simulink model "NewFSBER7f_1"  (Simulink 8.0)
settings: Solver=ode45  StartTime=0.0  StopTime=SystemSettings.SimEndTime  RelTol=1e-3
undefined symbols (not defined in the file): ChannelSettings, dfilt, outputcontrol, ShaperSettings, SystemSettings
libraries: dspmathops x14, dspsigattribs x10, dspsigops x9, simulink x5, dsparch4 x3, dspsrcs4 x3, commchan3 x1, commsink2 x1, commrandsrc2 x1
settings Model: Creator=cthomos  LastModifiedBy=Christos
settings DataIOCC: SignalLoggingSaveFormat=ModelDataLogs
settings OptimizationCC: InitFltsAndDblsToZero=on
settings DebuggingCC: SaveWithParameterizedLinksMsg=none  SignalResolutionControl=TryResolveAllWithWarning  FcnCallInpInsideContextMsg=UseLocalSettings  StrictBusMsg=Warning
settings GRTTargetCC: TargetFcnLib=ansi_tfl_tmw.mat  CombineOutputUpdateFcns=off  GRTInterface=on

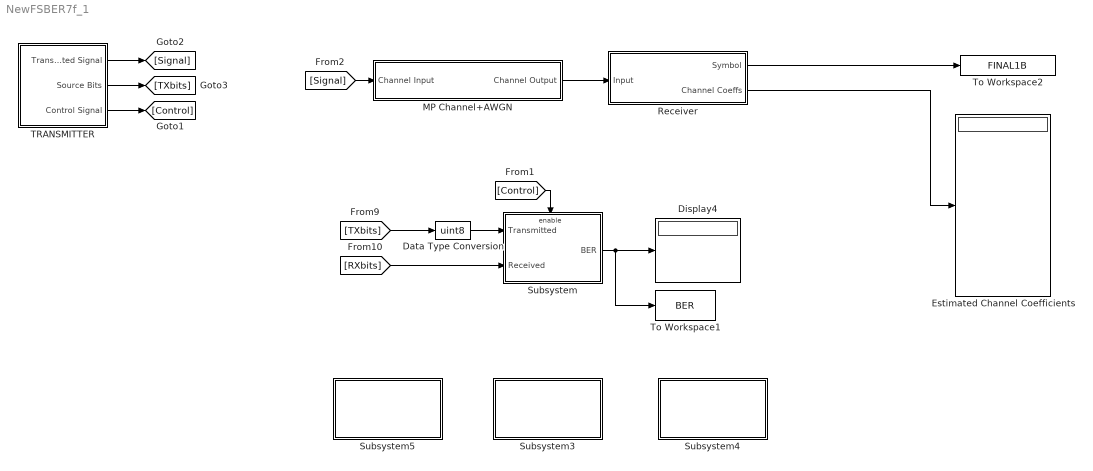
== system NewFSBER7f_1 ==
  Data Type Conversion : DataTypeConversion  OutDataTypeStr=uint8
  Display4 : Display
  Estimated Channel Coefficients : Display
  MP Channel+AWGN : Subsystem
  Receiver : Subsystem
  Subsystem : Subsystem
  Subsystem3 : Subsystem  mask(Pulse Shaper Settings){Tp=2e-9, pow=-30, Tpr=5e-9, GaussDrv=0, fc=50e9}
      mask prompts: Tp "Pulse Duration (sec)"; pow "Power (dBm):"; Tpr "Duration of a chip (sec):"; GaussDrv "Derivative Number"; fc "Sampling Frequency (Hz):"
      mask help: The parameters of this block determine the shape of the pulse to be used
      mask init:
      | ShaperSettings = PShaper_settings(...
      | 	Tp, ...
      | 	pow, ...
      | 	Tpr, ...
      | 	GaussDrv,...
      |     fc);
      | 
      | assignin('base', 'ShaperSettings', ShaperSettings);
      settings: AttributesFormatString="Pulse Duration = %<Tp> sec\\nPower = %<pow>  dBm\\nDerivative =  %<GaussDrv>\\nDuration of a chip = %<Tpr> sec\\nSampling Frequency = %<fc> Hz"
      mask Display: disp('Pulse Shaper\n Settings');
  Subsystem4 : Subsystem  mask(Set Channel Parameters){ChannelModel=CM1, UserDefined=Yes, tbin=5e-9, G2=on, fc=50e9}
      mask prompts: ChannelModel "Channel Model"; UserDefined "User Defined Channel"; tbin "Channel Resolution (sec)"; G2 "Graphical output"; fc "Sampling Frequency (Hz):"
      mask help:
      | % -------------------------------------------------------------------------
      | % ***** MULTIPATH CHANNEL ******
      | %--------------------------------------------------------------------------
      | % Initialization Commands of the multipath channel
      |
      | % 'ChannelModel' is one of the four scenarios:
      | % 'ChannelModel = 1' corresponds to Case A LOS (0-4m) CM1,
      | % 'ChannelModel = 2' corresponds to Case B NLOS (0-4m) CM2,
      | % 'ChannelModel = 3' corresponds to Case C NLOS (4-10m) CM3 and
      | % 'ChannelModel = 4' corresponds to Case D Extreme NLOS Multipath channel CM4.
      mask init:
      | ChannelSettings = MPChannel_settings(...
      | 	ChannelModel, ...
      | 	UserDefined, ...
      | 	tbin, ...
      | 	G2,...
      |     fc);
      | 
      | assignin('base', 'ChannelSettings', ChannelSettings);
      settings: AttributesFormatString=Channel Model = %<ChannelModel>\nUser Defined Channel = %<UserDefined>\nChannel Resolution (sec) = %<tbin>\nGraphical Output = %<G2>\nSampling Frequency = %<fc>
      mask TypeOptions ChannelModel: CM1 | CM2 | CM3 | CM4
      mask TypeOptions UserDefined: Yes | No
      mask Callback UserDefined:
      | if strcmp(get_param(gcb,'UserDefined'),'Yes')
      | 	set_param(gcb,'MaskEnables',{'off' 'on' 'off' 'on' 'off'})
      | else
      | 	set_param(gcb,'MaskEnables',{'on' 'on' 'on' 'on' 'on'})
      | end
      mask Display: disp('Multipath Channel\n Settings');
  Subsystem5 : Subsystem  mask{nBits=9, PNseq=[1 1 1 -1 1 -1 -1], fc=50e9, Tpr=5e-9, PayL=4, PilL=3}
      mask prompts: nBits "Number of bits to simulate:"; PNseq "PN Sequence:"; fc "System Sampling Frequency (Hz):"; Tpr "Duration of a chip (sec):"; PayL "Payload Length (bits):"; PilL "Pilot Length (bits):"
      mask init:
      | SystemSettings = System_settings(...
      | 	nBits, ...
      | 	PNseq, ...
      | 	fc, ...
      | 	Tpr,...
      |     PayL,...
      |     PilL);
      | 
      | assignin('base', 'SystemSettings', SystemSettings);
      settings: AttributesFormatString=Number of simulated bits = %<nBits>\nPN Sequence =\n%<PNseq>\nSampling Frequency = %<fc> Hz\nDuration of a chip = %<Tpr> sec\nPayload Length = %<PayL> bits\nPilot Length = %<PilL> bits
      mask Display: disp('Simulation\nSettings');
  TRANSMITTER : Subsystem
  To Workspace1 : ToWorkspace  VariableName=BER  SampleTime=-1
      settings: MaxDataPoints=1
  To Workspace2 : ToWorkspace  VariableName=FINAL1B  SampleTime=-1
  wires:
  TRANSMITTER/1(Transmitted Signal) -> [Signal]
  MP Channel+AWGN/1(Channel Output) -> Receiver/1(Input)
  TRANSMITTER/2(Source Bits) -> [TXbits]
  Receiver/1(Symbol) -> To Workspace2/1
  Receiver/2(Channel Coeffs) -> Estimated Channel Coefficients/1
  TRANSMITTER/3(Control Signal) -> [Control]
  [RXbits] -> Subsystem/2(Received)
  Subsystem/1(BER) -> Display4/1, To Workspace1/1
  [TXbits] -> Data Type Conversion/1
  Data Type Conversion/1 -> Subsystem/1(Transmitted)
  [Control] -> Subsystem/Enable
  [Signal] -> MP Channel+AWGN/1(Channel Input)

== system NewFSBER7f_1/MP Channel+AWGN ==
  Channel Input : Inport
  IEEE 802.15.3a Channel Model : Subsystem  mask(IEEE802.15.3a Channel Model){}
      mask help:
      | Channel choices are
      | CM1             IEEE line of sight, < 4m
      | CM2             IEEE non-line of sight, < 4m
      | CM3             IEEE non-line of sight, 4-10m
      | CM4             IEEE strong dispersion, delay spread of 25 nsec.
      mask Help:
      | The IEEE Multipath Channel block simulates an indoor UWB channel as described in "A Channel Model for Ultrawideband Indoor Communications" by J.R. Foerster, M. Pendergrass and A.F. Molisch, November 2003 and attempts to incorporate the processes used in their Matlab scripts.
      | 
      | The discrete input is convolved with a realization of the channel impulse response.  This response can be one of 4 types (CM1, CM2, CM3 or CM4) described in the paper or a custom channel with user-defined parameters.  A new channel realization is generated every symbol period.  Response terms that extend beyond one symbol period (ISI) are added to the output for the next symbol period.
      | 
      | Sample time is the rate at which the discrete signal is processed through the channel.  It represents the time resolution of the channel and is entered in nsec.  The symbol period is the time period of each data symbol and is entered as an integral number of sample times.  For example, enter
      | Sample Time:  0.02
      | Symbol Period:  100
      | for a signal with a symbol period of 2 nsec. and a sampling period of 20 psec.
      | 
      | Channel choices are
      | CM1             IEEE line of sight, < 4m
      | CM2             IEEE non-line of sight, < 4m
      | CM3             IEEE non-line of sight, 4-10m
      | CM4             IEEE strong dispersion, delay spread of 25 nsec.
      | custom         define parameters manually
      mask Display:
      | plot([.1 .9],[0.1 0.1]);
      | plot([.1 .1],[0.1 .8]);
      | plot([.23 .23],[0.1 .35]);
      | plot([.3 .3],[0.1 .65]);
      | plot([.4 .4],[0.1 .2]);
      | plot([.55 .55],[0.1 0.3]);
      | plot([.7 .7],[0.1 .15]);
      | plot([.85 .85],[0.1 0.18]);
  Subsystem1 : Subsystem  mask{exno=10000000, sChip=SystemSettings.SamplesPerChip, wtx=ShaperSettings.FinalPulseWaveform, attn=ChannelSettings.Attenuation}
      mask prompts: exno "Signal to Noise Ratio (Ex/No) (dB):"; sChip "Samples Per Chip:"; wtx "Pulse Waveform:"; attn "Attenuation of the MP channel:"
      mask init:
      | %--------------------------------------------------------------------------
      | % COMPUTATION OF THE NOISE VARIANCE
      | %--------------------------------------------------------------------------
      | 
      | % Create an impulse of length sChip
      | Impulse = [1, zeros(1,sChip-1)];
      | 
      | % Output of a shaping filter
      | Sa = conv(Impulse, wtx);
      | 
      | % Trim off the samples in excess originating from the convolution
      | L = sChip;
      | Stx = Sa(1:L);
      | 
      | % attenuation of the transmitted pulse
      | SRX0 = Stx.*attn;
      | 
      | % measured energy per pulse
      | Ex = sum(SRX0.^2);
      | 
      | % Ex/No in linear units
      | ExNoR = 10.^(exno./10);
      | 
      | % Unilateral spectral density
      | No = Ex./ExNoR;
      | 
      | % Noise Variance
      | noise_variance = No./2;
      | 
      | assignin('base','NoiseVariance',noise_variance);
      | 
      | % Noise Standard Deviation 
      | nstdv = sqrt(No./2);
      mask Display: disp('AWGN')
  Channel Output : Outport
  wires:
  IEEE 802.15.3a Channel Model/1(Out1) -> Subsystem1/1(In1)
  Channel Input/1 -> IEEE 802.15.3a Channel Model/1(In1)
  Subsystem1/1(Out1) -> Channel Output/1

== system NewFSBER7f_1/Receiver ==
  Input : Inport
  Channel Estimator and  Rake Receiver : Subsystem
      mask Display: disp('Channel Estimator\n Rake Receiver\n Simulink Comps');
  Downsample : dspsigops/Downsample  N=SystemSettings.SamplesPerChip  phase=ShaperSettings.NSPP  InputProcessing=Inherited (this choice will be removed - see release notes)  RateOptions=Enforce single-rate processing  smode=Allow multirate  fmode=Maintain input frame size  ic=0
  Gain : Gain  Gain=1/SystemSettings.SamplesPerChip*1e6
  Matched Filter : dsparch4/Digital Filter  TypePopup=FIR (all zeros)  IIRFiltStruct=Direct form II transposed  AllPoleFiltStruct=Direct form  FIRFiltStruct=Direct form  CoeffSource=Specify via dialog  NumCoeffs=ShaperSettings.MatchedPulseWaveform  DenCoeffs=1  BiQuadCoeffs=[1 0.3 0.4 1 0.1 0.2]  LatticeCoeffs=[0.2 0.4]  denIgnore=on  FiltPerSampPopup=One filter per frame  IC=0  ICnum=0  ICden=0  roundingMode=Floor  overflowMode=off  ScaleValues=1  scaleValueFracLength=14  stageInFracLength=15  stageOutFracLength=15  FilterSource=Specify via dialog  dfiltObjectName=dfilt.dffir([1 2 1])  InputProcessing=Inherited (this choice will be removed - see release notes)
  Symbol : Outport
  Channel Coeffs : Outport  Port=2
  wires:
  Gain/1 -> Downsample/1
  Matched Filter/1 -> Gain/1
  Downsample/1 -> Channel Estimator and  Rake Receiver/1(Input Signal)
  Channel Estimator and  Rake Receiver/1(Channel Coeeffs) -> Channel Coeffs/1
  Input/1 -> Matched Filter/1
  Channel Estimator and  Rake Receiver/2(FinalSymbol) -> Symbol/1

== system NewFSBER7f_1/Subsystem ==
  Transmitted : Inport
  Received : Inport  Port=2
  Enable : EnablePort  StatesWhenEnabling=reset
  Error Rate Calculation4 : commsink2/Error Rate Calculation  N=3  st_delay=0  cp_mode=Entire frame  subframe=[]  PMode=Port  WsName=ErrorVec  RsMode2=off  stop=on  numErr=100  maxBits=1e8
  BER : Outport
  wires:
  Transmitted/1 -> Error Rate Calculation4/1
  Error Rate Calculation4/1 -> BER/1
  Received/1 -> Error Rate Calculation4/2

== system NewFSBER7f_1/Subsystem3 ==
  note: This subsystem is empty.
      | It is used for setting parameter values (in the mask).

== system NewFSBER7f_1/Subsystem4 ==
  note: THIS SUBSYSTEM IS EMPTY

== system NewFSBER7f_1/Subsystem5 ==
  note: This subsystem is empty.
      | It is used for setting parameter values (in the mask).

== system NewFSBER7f_1/TRANSMITTER ==
  Pulse Shaper 2 : Subsystem  mask(UWB Gaussian Pulse Shaper){PulseShape=ShaperSettings.FinalPulseWaveform, Upsample=SystemSettings.SamplesPerChip}
      mask prompts: PulseShape "Filter Coeeficients for the Pulse Shaper:"; Upsample "Pulse Shaper Upsampling Factor:"
      mask Display:
      | plot(1:length(PulseShape), PulseShape);
      | disp('Pulse\n Shaper');
  Subsystem1 : Subsystem
      mask Display: disp('Pilot Signal');
  Subsystem4 : Subsystem
      mask Display: disp('Usefull Signal');
  Sum1 : Sum
  Transmission Control : DiscretePulseGenerator  Period=SystemSettings.ChipsPerBit*SystemSettings.FrameLength  PulseWidth=SystemSettings.ChipsPerBit*SystemSettings.UsefulDataL  PhaseDelay=SystemSettings.ChipsPerBit*SystemSettings.PilotLength  SampleTime=SystemSettings.ChipDuration
  Transmitted Signal : Outport
  Source Bits : Outport  Port=2
  Control Signal : Outport  Port=3
  wires:
  Subsystem4/2(Bits from Source) -> Source Bits/1
  Subsystem4/1(Usefull Signal) -> Sum1/2
  Subsystem1/1(Pilot Signal) -> Sum1/1
  Sum1/1 -> Pulse Shaper 2/1(In1)
  Transmission Control/1 -> Subsystem1/1(Control Signal), Subsystem4/1(Control Signal), Control Signal/1
  Pulse Shaper 2/1(Out1) -> Transmitted Signal/1

== system NewFSBER7f_1/MP Channel+AWGN/IEEE 802.15.3a Channel Model ==
  In1 : Inport
  Digital Filter : dsparch4/Digital Filter  TypePopup=FIR (all zeros)  IIRFiltStruct=Direct form II transposed  AllPoleFiltStruct=Direct form  FIRFiltStruct=Direct form  CoeffSource=Specify via dialog  NumCoeffs=ChannelSettings.ImpulseResponse  DenCoeffs=[1 0.1]  BiQuadCoeffs=[1 0.3 0.4 1 0.1 0.2]  LatticeCoeffs=[0.2 0.4]  denIgnore=on  FiltPerSampPopup=One filter per frame  IC=0  ICnum=0  ICden=0  roundingMode=Floor  overflowMode=off  ScaleValues=1  scaleValueFracLength=14  stageInFracLength=15  stageOutFracLength=15  FilterSource=Specify via dialog  dfiltObjectName=dfilt.dffir([1 2 1])
  Out1 : Outport
  wires:
  In1/1 -> Digital Filter/1
  Digital Filter/1 -> Out1/1

== system NewFSBER7f_1/MP Channel+AWGN/Subsystem1 ==
  In1 : Inport
  AWGN Channel : commchan3/AWGN Channel  SystemSampleTime=-1  seed=67  noiseMode=Variance from port  EbNodB=10  EsNodB=10  SNRdB=10  bitsPerSym=1  Ps=1  Tsym=1  variance=1
  Constant1 : Constant  Value=noise_variance
  Out1 : Outport
  wires:
  Constant1/1 -> AWGN Channel/2
  In1/1 -> AWGN Channel/1
  AWGN Channel/1 -> Out1/1

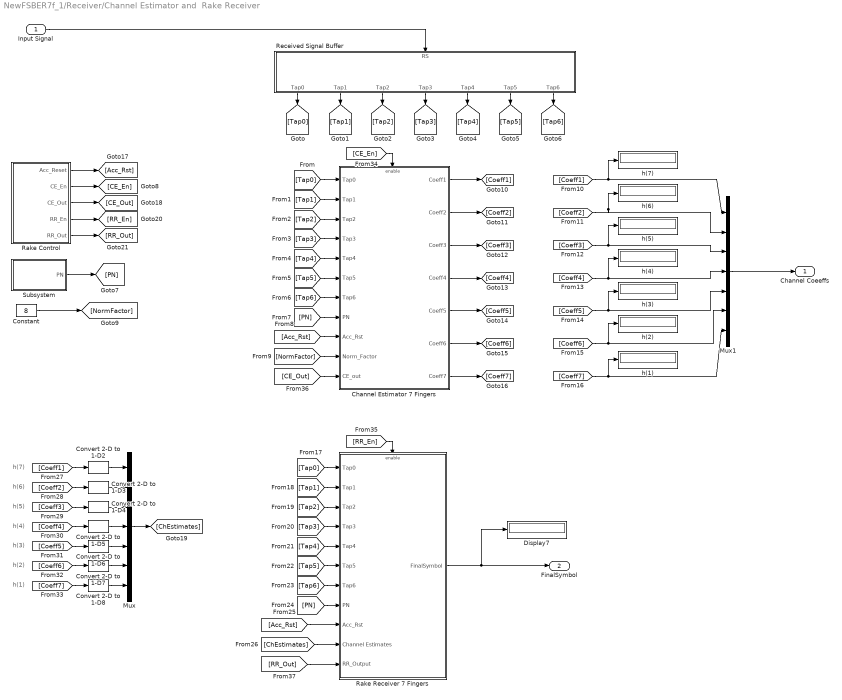
== system NewFSBER7f_1/Receiver/Channel Estimator and  Rake Receiver ==
  note: h(7)
  note: h(6)
  note: h(5)
  note: h(4)
  note: h(3)
  note: h(2)
  note: h(1)
  Input Signal : Inport
  Channel Estimator 7 Fingers : Subsystem
  Constant : Constant  Value=8
  Convert 2-D to 1-D{2..8} (7 alike) : dspsigattribs/Convert 2-D to 1-D
  Display7 : Display
  Mux : Mux  Inputs=7
  Mux1 : Mux  Inputs=7
  Rake Control : Subsystem
  Rake Receiver 7 Fingers : Subsystem
  Received Signal Buffer : Subsystem
  Subsystem : Subsystem
      mask Display: disp('PN Buffer');
  h(1) : Display
  h(2) : Display
  h(3) : Display
  h(4) : Display
  h(5) : Display
  h(6) : Display
  h(7) : Display
  Channel Coeeffs : Outport
  FinalSymbol : Outport  Port=2
  wires:
  Input Signal/1 -> Received Signal Buffer/1(RS)
  Received Signal Buffer/1(Tap0) -> [Tap0]
  Received Signal Buffer/2(Tap1) -> [Tap1]
  Received Signal Buffer/3(Tap2) -> [Tap2]
  Received Signal Buffer/4(Tap3) -> [Tap3]
  Received Signal Buffer/5(Tap4) -> [Tap4]
  Received Signal Buffer/6(Tap5) -> [Tap5]
  Received Signal Buffer/7(Tap6) -> [Tap6]
  Subsystem/1(PN) -> [PN]
  [Tap0] -> Channel Estimator 7 Fingers/1(Tap0)
  [Tap1] -> Channel Estimator 7 Fingers/2(Tap1)
  [Tap2] -> Channel Estimator 7 Fingers/3(Tap2)
  [Tap3] -> Channel Estimator 7 Fingers/4(Tap3)
  [Tap4] -> Channel Estimator 7 Fingers/5(Tap4)
  [Tap5] -> Channel Estimator 7 Fingers/6(Tap5)
  [Tap6] -> Channel Estimator 7 Fingers/7(Tap6)
  [PN] -> Channel Estimator 7 Fingers/8(PN)
  [Acc_Rst] -> Channel Estimator 7 Fingers/9(Acc_Rst)
  Constant/1 -> [NormFactor]
  [NormFactor] -> Channel Estimator 7 Fingers/10(Norm_Factor)
  Channel Estimator 7 Fingers/1(Coeff1) -> [Coeff1]
  Channel Estimator 7 Fingers/2(Coeff2) -> [Coeff2]
  Channel Estimator 7 Fingers/3(Coeff3) -> [Coeff3]
  Channel Estimator 7 Fingers/4(Coeff4) -> [Coeff4]
  Channel Estimator 7 Fingers/5(Coeff5) -> [Coeff5]
  Channel Estimator 7 Fingers/6(Coeff6) -> [Coeff6]
  Channel Estimator 7 Fingers/7(Coeff7) -> [Coeff7]
  [Coeff1] -> h(7)/1, Mux1/1
  [Coeff2] -> h(6)/1, Mux1/2
  [Coeff3] -> h(5)/1, Mux1/3
  [Coeff4] -> h(4)/1, Mux1/4
  [Coeff5] -> h(3)/1, Mux1/5
  [Coeff6] -> h(2)/1, Mux1/6
  [Coeff7] -> h(1)/1, Mux1/7
  [Tap0] -> Rake Receiver 7 Fingers/1(Tap0)
  [Tap1] -> Rake Receiver 7 Fingers/2(Tap1)
  [Tap2] -> Rake Receiver 7 Fingers/3(Tap2)
  [Tap3] -> Rake Receiver 7 Fingers/4(Tap3)
  [Tap4] -> Rake Receiver 7 Fingers/5(Tap4)
  [Tap5] -> Rake Receiver 7 Fingers/6(Tap5)
  [Tap6] -> Rake Receiver 7 Fingers/7(Tap6)
  [PN] -> Rake Receiver 7 Fingers/8(PN)
  [Acc_Rst] -> Rake Receiver 7 Fingers/9(Acc_Rst)
  [ChEstimates] -> Rake Receiver 7 Fingers/10(Channel Estimates)
  Rake Receiver 7 Fingers/1(FinalSymbol) -> Display7/1, FinalSymbol/1
  Convert 2-D to 1-D2/1 -> Mux/1
  Convert 2-D to 1-D3/1 -> Mux/2
  Convert 2-D to 1-D4/1 -> Mux/3
  Convert 2-D to 1-D5/1 -> Mux/4
  Convert 2-D to 1-D6/1 -> Mux/5
  Convert 2-D to 1-D7/1 -> Mux/6
  Mux/1 -> [ChEstimates]
  Convert 2-D to 1-D8/1 -> Mux/7
  Rake Control/1(Acc_Reset) -> [Acc_Rst]
  [Coeff1] -> Convert 2-D to 1-D2/1
  [Coeff2] -> Convert 2-D to 1-D3/1
  [Coeff3] -> Convert 2-D to 1-D4/1
  [Coeff4] -> Convert 2-D to 1-D5/1
  [Coeff5] -> Convert 2-D to 1-D6/1
  [Coeff6] -> Convert 2-D to 1-D7/1
  [Coeff7] -> Convert 2-D to 1-D8/1
  Rake Control/2(CE_En) -> [CE_En]
  Rake Control/3(CE_Out) -> [CE_Out]
  Rake Control/4(RR_En) -> [RR_En]
  Rake Control/5(RR_Out) -> [RR_Out]
  [CE_En] -> Channel Estimator 7 Fingers/Enable
  [RR_En] -> Rake Receiver 7 Fingers/Enable
  [CE_Out] -> Channel Estimator 7 Fingers/11(CE_out)
  [RR_Out] -> Rake Receiver 7 Fingers/11(RR_Output)
  Mux1/1 -> Channel Coeeffs/1

== system NewFSBER7f_1/TRANSMITTER/Pulse Shaper 2 ==
  In1 : Inport
  Pulse Shaping Filter : dsparch4/Digital Filter  TypePopup=FIR (all zeros)  IIRFiltStruct=Direct form II transposed  AllPoleFiltStruct=Direct form  FIRFiltStruct=Direct form  CoeffSource=Specify via dialog  NumCoeffs=PulseShape  DenCoeffs=1  BiQuadCoeffs=[1 0.3 0.4 1 0.1 0.2]  LatticeCoeffs=[0.2 0.4]  denIgnore=on  FiltPerSampPopup=One filter per frame  IC=0  ICnum=0  ICden=0  roundingMode=Floor  overflowMode=off  ScaleValues=1  scaleValueFracLength=14  stageInFracLength=15  stageOutFracLength=15  FilterSource=Specify via dialog  dfiltObjectName=dfilt.dffir([1 2 1])
  Upsample : dspsigops/Upsample  N=Upsample  phase=0  ic=0  mode=Maintain input frame size
  Out1 : Outport
  wires:
  Upsample/1 -> Pulse Shaping Filter/1
  Pulse Shaping Filter/1 -> Out1/1
  In1/1 -> Upsample/1

== system NewFSBER7f_1/TRANSMITTER/Subsystem1 ==
  Control Signal : Inport
  Convert 2-D to 1-D1 : dspsigattribs/Convert 2-D to 1-D  SystemSampleTime=-1
  Logical Operator : Logic  Operator=NOT  Inputs=1  AllPortsSameDT=off  OutDataTypeStr=boolean
  PNsequence : dspsrcs4/Signal From Workspace  SystemSampleTime=-1  X=SystemSettings.PNSequence  Ts=SystemSettings.ChipDuration  nsamps=1  OutputAfterFinalValue=Cyclic repetition  ignoreOrWarnInputAndFrameLengths=off
  Spreading : Product  RndMeth=Zero
  Pilot Signal : Outport
  wires:
  Control Signal/1 -> Logical Operator/1
  Spreading/1 -> Pilot Signal/1
  PNsequence/1 -> Convert 2-D to 1-D1/1
  Convert 2-D to 1-D1/1 -> Spreading/2
  Logical Operator/1 -> Spreading/1

== system NewFSBER7f_1/TRANSMITTER/Subsystem4 ==
  Control Signal : Inport
  Convert 2-D to 1-D1 : dspsigattribs/Convert 2-D to 1-D  SystemSampleTime=-1
  PNsequence : dspsrcs4/Signal From Workspace  SystemSampleTime=-1  X=SystemSettings.PNSequence  Ts=SystemSettings.ChipDuration  nsamps=1  OutputAfterFinalValue=Cyclic repetition  ignoreOrWarnInputAndFrameLengths=off
  Spreading : Product  Inputs=3  RndMeth=Zero
  Subsystem1 : Subsystem
      mask Display: disp('BPSK \n Modulation')
  Subsystem2 : Subsystem
      mask Display: disp('Bits Source')
  Usefull Signal : Outport
  Bits from Source : Outport  Port=2
  wires:
  Spreading/1 -> Usefull Signal/1
  PNsequence/1 -> Convert 2-D to 1-D1/1
  Control Signal/1 -> Subsystem2/Enable, Spreading/2
  Subsystem2/1(Out1) -> Subsystem1/1(In1), Bits from Source/1
  Subsystem1/1(Out1) -> Spreading/3
  Convert 2-D to 1-D1/1 -> Spreading/1

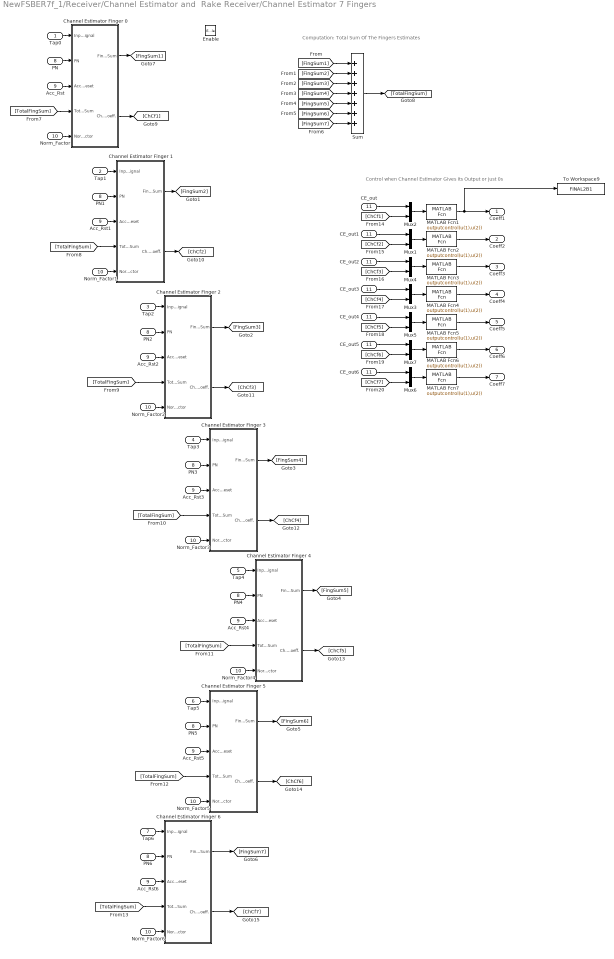
== system NewFSBER7f_1/Receiver/Channel Estimator and  Rake Receiver/Channel Estimator 7 Fingers ==
  note: Computation: Total Sum Of The Fingers Estimates
  note: Control when Channel Estimator Gives Its Output or just 0s
  Tap0 : Inport
  Tap1 : Inport  Port=2
  Tap2 : Inport  Port=3
  Tap3 : Inport  Port=4
  Tap4 : Inport  Port=5
  Tap5 : Inport  Port=6
  Tap6 : Inport  Port=7
  PN : Inport  Port=8
  Acc_Rst : Inport  Port=9
  Norm_Factor : Inport  Port=10
  CE_out : Inport  Port=11
  Enable : EnablePort  StatesWhenEnabling=reset
  Acc_Rst{1..6} (6 alike) : InportShadow  Port=9
  CE_out{1..6} (6 alike) : InportShadow  Port=11
  Channel Estimator Finger 0 : Subsystem
  Channel Estimator Finger 1 : Subsystem
  Channel Estimator Finger 2 : Subsystem
  Channel Estimator Finger 3 : Subsystem
  Channel Estimator Finger 4 : Subsystem
  Channel Estimator Finger 5 : Subsystem
  Channel Estimator Finger 6 : Subsystem
  MATLAB Fcn{1..7} (7 alike) : MATLABFcn  MATLABFcn=outputcontrol(u(1),u(2))
  Mux{1..7} (7 alike) : Mux  Inputs=2
  Norm_Factor{1..6} (6 alike) : InportShadow  Port=10
  PN{1..6} (6 alike) : InportShadow  Port=8
  Sum : Sum  Inputs=+++++++
  To Workspace9 : ToWorkspace  VariableName=FINAL2B1  SampleTime=-1
  Coeff1 : Outport
  Coeff2 : Outport  Port=2
  Coeff3 : Outport  Port=3
  Coeff4 : Outport  Port=4
  Coeff5 : Outport  Port=5
  Coeff6 : Outport  Port=6
  Coeff7 : Outport  Port=7
  wires:
  Tap0/1 -> Channel Estimator Finger 0/1(Input Signal)
  Tap1/1 -> Channel Estimator Finger 1/1(Input Signal)
  Tap2/1 -> Channel Estimator Finger 2/1(Input Signal)
  Tap3/1 -> Channel Estimator Finger 3/1(Input Signal)
  Tap4/1 -> Channel Estimator Finger 4/1(Input Signal)
  Tap6/1 -> Channel Estimator Finger 6/1(Input Signal)
  PN/1 -> Channel Estimator Finger 0/2(PN)
  PN1/1 -> Channel Estimator Finger 1/2(PN)
  PN2/1 -> Channel Estimator Finger 2/2(PN)
  PN3/1 -> Channel Estimator Finger 3/2(PN)
  PN4/1 -> Channel Estimator Finger 4/2(PN)
  PN5/1 -> Channel Estimator Finger 5/2(PN)
  PN6/1 -> Channel Estimator Finger 6/2(PN)
  Tap5/1 -> Channel Estimator Finger 5/1(Input Signal)
  Channel Estimator Finger 0/2(Ch. Coeff.) -> [ChCf1]
  Channel Estimator Finger 1/2(Ch. Coeff.) -> [ChCf2]
  Channel Estimator Finger 2/2(Ch. Coeff.) -> [ChCf3]
  Channel Estimator Finger 3/2(Ch. Coeff.) -> [ChCf4]
  Channel Estimator Finger 4/2(Ch. Coeff.) -> [ChCf5]
  Channel Estimator Finger 5/2(Ch. Coeff.) -> [ChCf6]
  Channel Estimator Finger 6/2(Ch. Coeff.) -> [ChCf7]
  Acc_Rst/1 -> Channel Estimator Finger 0/3(Acc Reset)
  Acc_Rst1/1 -> Channel Estimator Finger 1/3(Acc Reset)
  Acc_Rst2/1 -> Channel Estimator Finger 2/3(Acc Reset)
  Acc_Rst3/1 -> Channel Estimator Finger 3/3(Acc Reset)
  Acc_Rst4/1 -> Channel Estimator Finger 4/3(Acc Reset)
  Acc_Rst5/1 -> Channel Estimator Finger 5/3(Acc Reset)
  Acc_Rst6/1 -> Channel Estimator Finger 6/3(Acc Reset)
  Norm_Factor/1 -> Channel Estimator Finger 0/5(Norm Factor)
  Norm_Factor1/1 -> Channel Estimator Finger 1/5(Norm Factor)
  Norm_Factor2/1 -> Channel Estimator Finger 2/5(Norm Factor)
  Norm_Factor3/1 -> Channel Estimator Finger 3/5(Norm Factor)
  Norm_Factor4/1 -> Channel Estimator Finger 4/5(Norm Factor)
  Norm_Factor5/1 -> Channel Estimator Finger 5/5(Norm Factor)
  Norm_Factor6/1 -> Channel Estimator Finger 6/5(Norm Factor)
  Channel Estimator Finger 0/1(Finger Sum) -> [FingSum1]
  Channel Estimator Finger 1/1(Finger Sum) -> [FingSum2]
  Channel Estimator Finger 2/1(Finger Sum) -> [FingSum3]
  Channel Estimator Finger 3/1(Finger Sum) -> [FingSum4]
  Channel Estimator Finger 4/1(Finger Sum) -> [FingSum5]
  Channel Estimator Finger 5/1(Finger Sum) -> [FingSum6]
  Channel Estimator Finger 6/1(Finger Sum) -> [FingSum7]
  [FingSum1] -> Sum/1
  [FingSum2] -> Sum/2
  [FingSum3] -> Sum/3
  [FingSum4] -> Sum/4
  [FingSum5] -> Sum/5
  [FingSum6] -> Sum/6
  [FingSum7] -> Sum/7
  Sum/1 -> [TotalFingSum]
  [TotalFingSum] -> Channel Estimator Finger 0/4(Total Sum)
  [TotalFingSum] -> Channel Estimator Finger 1/4(Total Sum)
  [TotalFingSum] -> Channel Estimator Finger 2/4(Total Sum)
  [TotalFingSum] -> Channel Estimator Finger 3/4(Total Sum)
  [TotalFingSum] -> Channel Estimator Finger 4/4(Total Sum)
  [TotalFingSum] -> Channel Estimator Finger 5/4(Total Sum)
  [TotalFingSum] -> Channel Estimator Finger 6/4(Total Sum)
  MATLAB Fcn1/1 -> Coeff1/1, To Workspace9/1
  Mux2/1 -> MATLAB Fcn1/1
  MATLAB Fcn2/1 -> Coeff2/1
  Mux1/1 -> MATLAB Fcn2/1
  MATLAB Fcn3/1 -> Coeff3/1
  Mux4/1 -> MATLAB Fcn3/1
  MATLAB Fcn4/1 -> Coeff4/1
  Mux3/1 -> MATLAB Fcn4/1
  MATLAB Fcn5/1 -> Coeff5/1
  Mux5/1 -> MATLAB Fcn5/1
  MATLAB Fcn6/1 -> Coeff6/1
  Mux7/1 -> MATLAB Fcn6/1
  MATLAB Fcn7/1 -> Coeff7/1
  Mux6/1 -> MATLAB Fcn7/1
  [ChCf1] -> Mux2/2
  [ChCf2] -> Mux1/2
  [ChCf3] -> Mux4/2
  [ChCf4] -> Mux3/2
  [ChCf5] -> Mux5/2
  [ChCf6] -> Mux7/2
  [ChCf7] -> Mux6/2
  CE_out/1 -> Mux2/1
  CE_out1/1 -> Mux1/1
  CE_out2/1 -> Mux4/1
  CE_out3/1 -> Mux3/1
  CE_out4/1 -> Mux5/1
  CE_out5/1 -> Mux7/1
  CE_out6/1 -> Mux6/1

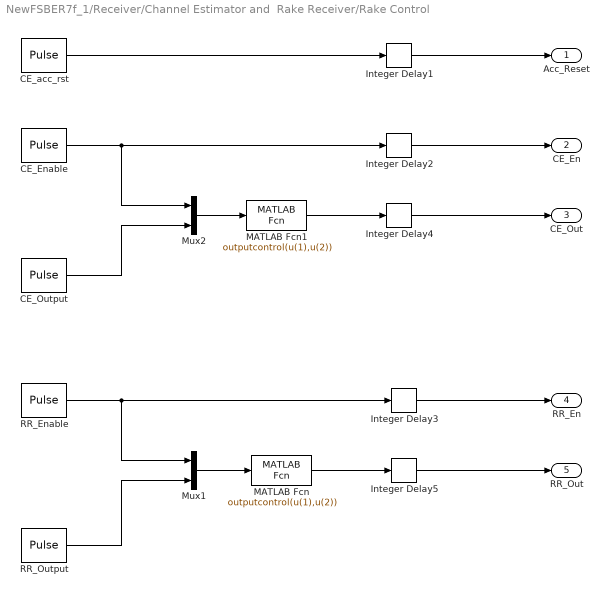
== system NewFSBER7f_1/Receiver/Channel Estimator and  Rake Receiver/Rake Control ==
  CE_Enable : DiscretePulseGenerator  Period=SystemSettings.ChipsPerBit*SystemSettings.FrameLength  PulseWidth=SystemSettings.ChipsPerBit  PhaseDelay=(SystemSettings.PilotLength-1)*SystemSettings.ChipsPerBit-1  SampleTime=SystemSettings.ChipDuration
  CE_Output : DiscretePulseGenerator  Period=SystemSettings.ChipsPerBit  PhaseDelay=SystemSettings.ChipsPerBit-2  SampleTime=SystemSettings.ChipDuration
  CE_acc_rst : DiscretePulseGenerator  Period=SystemSettings.ChipsPerBit  PhaseDelay=SystemSettings.ChipsPerBit-1  SampleTime=SystemSettings.ChipDuration
  Integer Delay{1..5} (5 alike) : simulink/Discrete/Integer Delay  vinit=0  samptime=-1  NumDelays=1
  MATLAB Fcn : MATLABFcn  MATLABFcn=outputcontrol(u(1),u(2))
  MATLAB Fcn1 : MATLABFcn  MATLABFcn=outputcontrol(u(1),u(2))
  Mux1 : Mux  Inputs=2
  Mux2 : Mux  Inputs=2
  RR_Enable : DiscretePulseGenerator  Period=SystemSettings.ChipsPerBit*SystemSettings.FrameLength+SystemSettings.ChipsPerBit-1  PulseWidth=SystemSettings.ChipsPerBit*SystemSettings.UsefulDataL  PhaseDelay=SystemSettings.PilotLength*SystemSettings.ChipsPerBit+SystemSettings.ChipsPerBit-1  SampleTime=SystemSettings.ChipDuration
  RR_Output : DiscretePulseGenerator  Period=SystemSettings.ChipsPerBit  PhaseDelay=SystemSettings.ChipsPerBit-2  SampleTime=SystemSettings.ChipDuration
  Acc_Reset : Outport
  CE_En : Outport  Port=2
  CE_Out : Outport  Port=3
  RR_En : Outport  Port=4
  RR_Out : Outport  Port=5
  wires:
  CE_acc_rst/1 -> Integer Delay1/1
  CE_Enable/1 -> Integer Delay2/1, Mux2/1
  CE_Output/1 -> Mux2/2
  RR_Enable/1 -> Mux1/1, Integer Delay3/1
  RR_Output/1 -> Mux1/2
  Mux1/1 -> MATLAB Fcn/1
  MATLAB Fcn/1 -> Integer Delay5/1
  Integer Delay1/1 -> Acc_Reset/1
  Integer Delay2/1 -> CE_En/1
  Mux2/1 -> MATLAB Fcn1/1
  MATLAB Fcn1/1 -> Integer Delay4/1
  Integer Delay4/1 -> CE_Out/1
  Integer Delay3/1 -> RR_En/1
  Integer Delay5/1 -> RR_Out/1

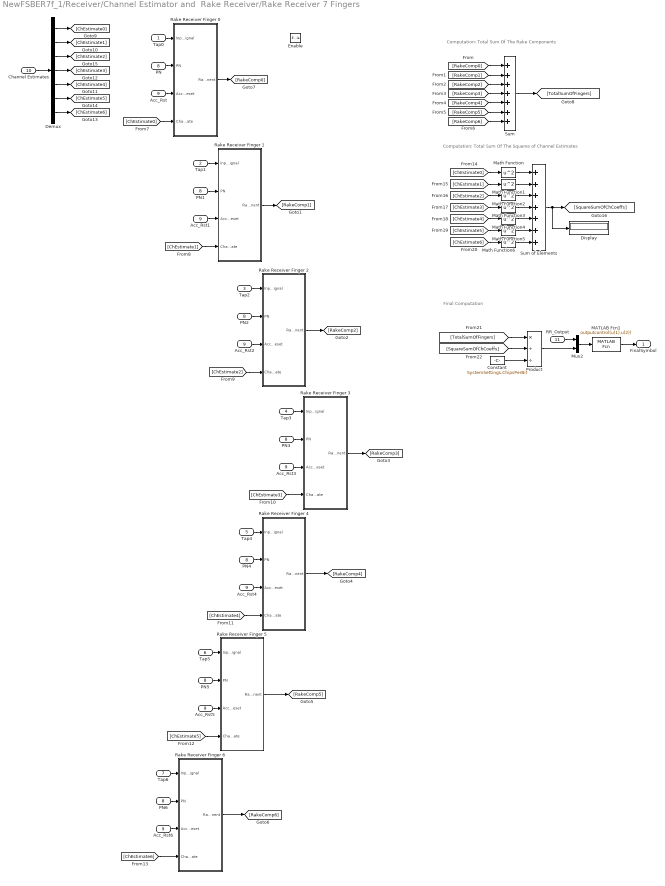
== system NewFSBER7f_1/Receiver/Channel Estimator and  Rake Receiver/Rake Receiver 7 Fingers ==
  note: Computation: Total Sum Of The Rake Components
  note: Computation: Total Sum Of The Squares of Channel Estimates
  note: Final Computation
  Tap0 : Inport
  Tap1 : Inport  Port=2
  Tap2 : Inport  Port=3
  Tap3 : Inport  Port=4
  Tap4 : Inport  Port=5
  Tap5 : Inport  Port=6
  Tap6 : Inport  Port=7
  PN : Inport  Port=8
  Acc_Rst : Inport  Port=9
  Channel Estimates : Inport  Port=10
  RR_Output : Inport  Port=11
  Enable : EnablePort  StatesWhenEnabling=reset
  Acc_Rst{1..6} (6 alike) : InportShadow  Port=9
  Constant : Constant  Value=SystemSettings.ChipsPerBit
  Demux : Demux  Outputs=7
  Display : Display
  MATLAB Fcn1 : MATLABFcn  MATLABFcn=outputcontrol(u(1),u(2))
  Math Function{,1..6} (7 alike) : Math  Operator=square  SaturateOnIntegerOverflow=on
  Mux2 : Mux  Inputs=2
  PN{1..6} (6 alike) : InportShadow  Port=8
  Product : Product  Inputs=*//  RndMeth=Zero
  Rake Receiver Finger 0 : Subsystem
  Rake Receiver Finger 1 : Subsystem
  Rake Receiver Finger 2 : Subsystem
  Rake Receiver Finger 3 : Subsystem
  Rake Receiver Finger 4 : Subsystem
  Rake Receiver Finger 5 : Subsystem
  Rake Receiver Finger 6 : Subsystem
  Sum : Sum  Inputs=+++++++
  Sum of Elements : Sum  Inputs=+++++++
  FinalSymbol : Outport
  wires:
  Tap0/1 -> Rake Receiver Finger 0/1(Input Signal)
  PN/1 -> Rake Receiver Finger 0/2(PN)
  Rake Receiver Finger 0/1(Rake Component) -> [RakeComp0]
  Acc_Rst/1 -> Rake Receiver Finger 0/3(Acc Reset)
  [ChEstimate0] -> Rake Receiver Finger 0/4(Channel Estimate)
  [RakeComp0] -> Sum/1
  [RakeComp1] -> Sum/2
  [RakeComp2] -> Sum/3
  [RakeComp3] -> Sum/4
  [RakeComp4] -> Sum/5
  [RakeComp5] -> Sum/6
  [RakeComp6] -> Sum/7
  Sum/1 -> [TotalSumOfFingers]
  Channel Estimates/1 -> Demux/1
  Demux/1 -> [ChEstimate0]
  Demux/2 -> [ChEstimate1]
  Demux/3 -> [ChEstimate2]
  Demux/4 -> [ChEstimate3]
  Demux/5 -> [ChEstimate4]
  Demux/6 -> [ChEstimate5]
  Demux/7 -> [ChEstimate6]
  Rake Receiver Finger 1/1(Rake Component) -> [RakeComp1]
  Rake Receiver Finger 2/1(Rake Component) -> [RakeComp2]
  Rake Receiver Finger 3/1(Rake Component) -> [RakeComp3]
  Rake Receiver Finger 4/1(Rake Component) -> [RakeComp4]
  Rake Receiver Finger 5/1(Rake Component) -> [RakeComp5]
  Rake Receiver Finger 6/1(Rake Component) -> [RakeComp6]
  Tap1/1 -> Rake Receiver Finger 1/1(Input Signal)
  Tap2/1 -> Rake Receiver Finger 2/1(Input Signal)
  Tap3/1 -> Rake Receiver Finger 3/1(Input Signal)
  Tap4/1 -> Rake Receiver Finger 4/1(Input Signal)
  Tap5/1 -> Rake Receiver Finger 5/1(Input Signal)
  Tap6/1 -> Rake Receiver Finger 6/1(Input Signal)
  PN1/1 -> Rake Receiver Finger 1/2(PN)
  PN2/1 -> Rake Receiver Finger 2/2(PN)
  PN3/1 -> Rake Receiver Finger 3/2(PN)
  PN4/1 -> Rake Receiver Finger 4/2(PN)
  PN5/1 -> Rake Receiver Finger 5/2(PN)
  PN6/1 -> Rake Receiver Finger 6/2(PN)
  Acc_Rst1/1 -> Rake Receiver Finger 1/3(Acc Reset)
  Acc_Rst2/1 -> Rake Receiver Finger 2/3(Acc Reset)
  Acc_Rst3/1 -> Rake Receiver Finger 3/3(Acc Reset)
  Acc_Rst4/1 -> Rake Receiver Finger 4/3(Acc Reset)
  Acc_Rst5/1 -> Rake Receiver Finger 5/3(Acc Reset)
  Acc_Rst6/1 -> Rake Receiver Finger 6/3(Acc Reset)
  [ChEstimate1] -> Rake Receiver Finger 1/4(Channel Estimate)
  [ChEstimate2] -> Rake Receiver Finger 2/4(Channel Estimate)
  [ChEstimate3] -> Rake Receiver Finger 3/4(Channel Estimate)
  [ChEstimate4] -> Rake Receiver Finger 4/4(Channel Estimate)
  [ChEstimate5] -> Rake Receiver Finger 5/4(Channel Estimate)
  [ChEstimate6] -> Rake Receiver Finger 6/4(Channel Estimate)
  [ChEstimate0] -> Math Function/1
  Math Function/1 -> Sum of Elements/1
  [ChEstimate1] -> Math Function1/1
  Math Function1/1 -> Sum of Elements/2
  [ChEstimate2] -> Math Function2/1
  Math Function2/1 -> Sum of Elements/3
  [ChEstimate3] -> Math Function3/1
  Math Function3/1 -> Sum of Elements/4
  [ChEstimate4] -> Math Function4/1
  Math Function4/1 -> Sum of Elements/5
  [ChEstimate5] -> Math Function5/1
  Math Function5/1 -> Sum of Elements/6
  [ChEstimate6] -> Math Function6/1
  Math Function6/1 -> Sum of Elements/7
  Sum of Elements/1 -> [SquareSumOfChCoeffs], Display/1
  MATLAB Fcn1/1 -> FinalSymbol/1
  Mux2/1 -> MATLAB Fcn1/1
  Product/1 -> Mux2/2
  RR_Output/1 -> Mux2/1
  [TotalSumOfFingers] -> Product/1
  [SquareSumOfChCoeffs] -> Product/2
  Constant/1 -> Product/3

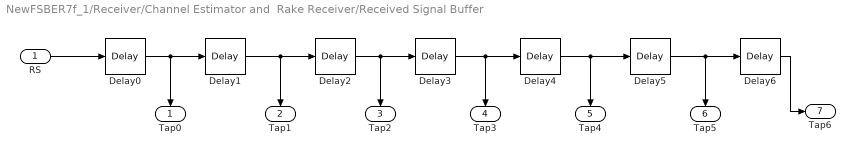
== system NewFSBER7f_1/Receiver/Channel Estimator and  Rake Receiver/Received Signal Buffer ==
  RS : Inport
  Delay0 : dspsigops/Delay  dly_unit=Samples  delay=0  ic_detail=off  dif_ic_for_ch=off  dif_ic_for_dly=off  ic=0  reset_popup=None
  Delay{1..6} (6 alike) : dspsigops/Delay  dly_unit=Samples  delay=1  ic_detail=off  dif_ic_for_ch=off  dif_ic_for_dly=off  ic=0  reset_popup=None
  Tap0 : Outport
  Tap1 : Outport  Port=2
  Tap2 : Outport  Port=3
  Tap3 : Outport  Port=4
  Tap4 : Outport  Port=5
  Tap5 : Outport  Port=6
  Tap6 : Outport  Port=7
  wires:
  Delay5/1 -> Delay6/1, Tap5/1
  Delay3/1 -> Delay4/1, Tap3/1
  Delay4/1 -> Delay5/1, Tap4/1
  Delay2/1 -> Delay3/1, Tap2/1
  Delay1/1 -> Delay2/1, Tap1/1
  Delay0/1 -> Delay1/1, Tap0/1
  Delay6/1 -> Tap6/1
  RS/1 -> Delay0/1

== system NewFSBER7f_1/Receiver/Channel Estimator and  Rake Receiver/Subsystem ==
  Convert 2-D to 1-D1 : dspsigattribs/Convert 2-D to 1-D  SystemSampleTime=-1
  Signal From Workspace6 : dspsrcs4/Signal From Workspace  SystemSampleTime=-1  X=SystemSettings.PNSequence  Ts=SystemSettings.ChipDuration  nsamps=1  OutputAfterFinalValue=Cyclic repetition  ignoreOrWarnInputAndFrameLengths=off
  PN : Outport
  wires:
  Signal From Workspace6/1 -> Convert 2-D to 1-D1/1
  Convert 2-D to 1-D1/1 -> PN/1

== system NewFSBER7f_1/TRANSMITTER/Subsystem4/Subsystem1 ==
  In1 : Inport
  Lookup Table : Lookup  InputValues=[0 1]  Table=[-1 +1]
  Out1 : Outport
  wires:
  Lookup Table/1 -> Out1/1
  In1/1 -> Lookup Table/1

== system NewFSBER7f_1/TRANSMITTER/Subsystem4/Subsystem2 ==
  Enable : EnablePort  StatesWhenEnabling=reset
  Random Integer Generator : commrandsrc2/Random Integer Generator  SystemSampleTime=-1  mul=2  seed=55  Ts=SystemSettings.BitDuration  frameBased=off  sampPerFrame=1  orient=off  outDataType=double
  Out1 : Outport
  wires:
  Random Integer Generator/1 -> Out1/1

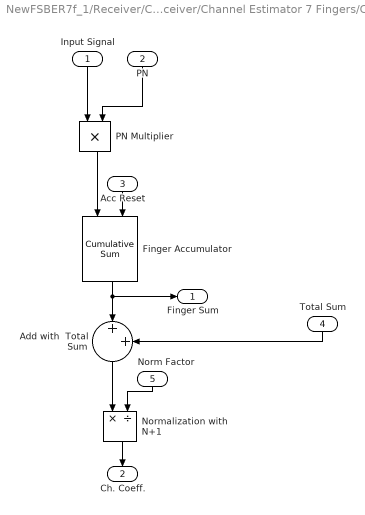
== system NewFSBER7f_1/Receiver/Channel Estimator and  Rake Receiver/Channel Estimator 7 Fingers/Channel Estimator Finger 0 ==
  Input Signal : Inport
  PN : Inport  Port=2
  Acc Reset : Inport  Port=3
  Total Sum : Inport  Port=4
  Norm Factor : Inport  Port=5
  Add with  Total Sum : Sum  Inputs=|++
  Finger Accumulator : dspmathops/Cumulative Sum  dim=Channels (running sum)  reset_popup=Rising edge  roundingMode=Floor  overflowMode=off
  Normalization with N+1 : Product  Inputs=*/
  PN Multiplier : Product  RndMeth=Zero
  Finger Sum : Outport
  Ch. Coeff. : Outport  Port=2
  wires:
  PN Multiplier/1 -> Finger Accumulator/1
  Finger Accumulator/1 -> Add with  Total Sum/1, Finger Sum/1
  Add with  Total Sum/1 -> Normalization with N+1/1
  Input Signal/1 -> PN Multiplier/1
  PN/1 -> PN Multiplier/2
  Acc Reset/1 -> Finger Accumulator/2
  Total Sum/1 -> Add with  Total Sum/2
  Norm Factor/1 -> Normalization with N+1/2
  Normalization with N+1/1 -> Ch. Coeff./1

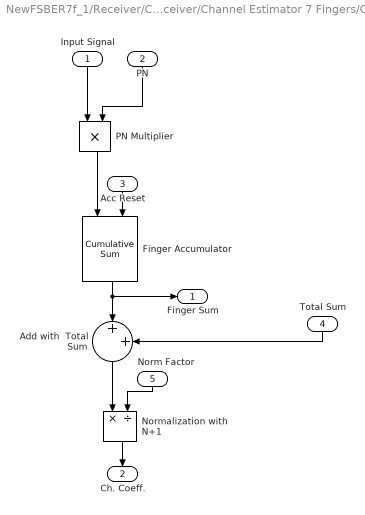
== system NewFSBER7f_1/Receiver/Channel Estimator and  Rake Receiver/Channel Estimator 7 Fingers/Channel Estimator Finger 1 ==
  Input Signal : Inport
  PN : Inport  Port=2
  Acc Reset : Inport  Port=3
  Total Sum : Inport  Port=4
  Norm Factor : Inport  Port=5
  Add with  Total Sum : Sum  Inputs=|++
  Finger Accumulator : dspmathops/Cumulative Sum  dim=Channels (running sum)  reset_popup=Rising edge  roundingMode=Floor  overflowMode=off
  Normalization with N+1 : Product  Inputs=*/
  PN Multiplier : Product  RndMeth=Zero
  Finger Sum : Outport
  Ch. Coeff. : Outport  Port=2
  wires:
  PN Multiplier/1 -> Finger Accumulator/1
  Finger Accumulator/1 -> Add with  Total Sum/1, Finger Sum/1
  Add with  Total Sum/1 -> Normalization with N+1/1
  Input Signal/1 -> PN Multiplier/1
  PN/1 -> PN Multiplier/2
  Acc Reset/1 -> Finger Accumulator/2
  Total Sum/1 -> Add with  Total Sum/2
  Norm Factor/1 -> Normalization with N+1/2
  Normalization with N+1/1 -> Ch. Coeff./1

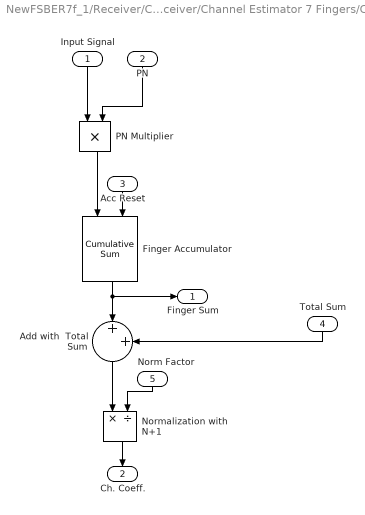
== system NewFSBER7f_1/Receiver/Channel Estimator and  Rake Receiver/Channel Estimator 7 Fingers/Channel Estimator Finger 2 ==
  Input Signal : Inport
  PN : Inport  Port=2
  Acc Reset : Inport  Port=3
  Total Sum : Inport  Port=4
  Norm Factor : Inport  Port=5
  Add with  Total Sum : Sum  Inputs=|++
  Finger Accumulator : dspmathops/Cumulative Sum  dim=Channels (running sum)  reset_popup=Rising edge  roundingMode=Floor  overflowMode=off
  Normalization with N+1 : Product  Inputs=*/
  PN Multiplier : Product  RndMeth=Zero
  Finger Sum : Outport
  Ch. Coeff. : Outport  Port=2
  wires:
  PN Multiplier/1 -> Finger Accumulator/1
  Finger Accumulator/1 -> Add with  Total Sum/1, Finger Sum/1
  Add with  Total Sum/1 -> Normalization with N+1/1
  Input Signal/1 -> PN Multiplier/1
  PN/1 -> PN Multiplier/2
  Acc Reset/1 -> Finger Accumulator/2
  Total Sum/1 -> Add with  Total Sum/2
  Norm Factor/1 -> Normalization with N+1/2
  Normalization with N+1/1 -> Ch. Coeff./1

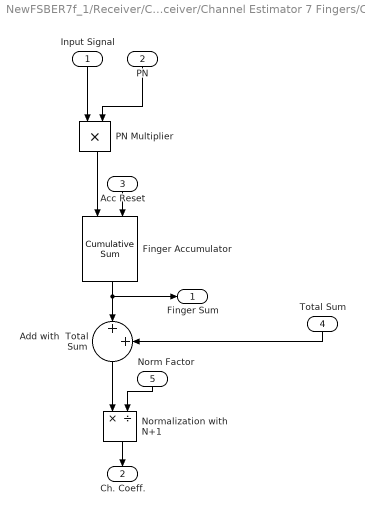
== system NewFSBER7f_1/Receiver/Channel Estimator and  Rake Receiver/Channel Estimator 7 Fingers/Channel Estimator Finger 3 ==
  Input Signal : Inport
  PN : Inport  Port=2
  Acc Reset : Inport  Port=3
  Total Sum : Inport  Port=4
  Norm Factor : Inport  Port=5
  Add with  Total Sum : Sum  Inputs=|++
  Finger Accumulator : dspmathops/Cumulative Sum  dim=Channels (running sum)  reset_popup=Rising edge  roundingMode=Floor  overflowMode=off
  Normalization with N+1 : Product  Inputs=*/
  PN Multiplier : Product  RndMeth=Zero
  Finger Sum : Outport
  Ch. Coeff. : Outport  Port=2
  wires:
  PN Multiplier/1 -> Finger Accumulator/1
  Finger Accumulator/1 -> Add with  Total Sum/1, Finger Sum/1
  Add with  Total Sum/1 -> Normalization with N+1/1
  Input Signal/1 -> PN Multiplier/1
  PN/1 -> PN Multiplier/2
  Acc Reset/1 -> Finger Accumulator/2
  Total Sum/1 -> Add with  Total Sum/2
  Norm Factor/1 -> Normalization with N+1/2
  Normalization with N+1/1 -> Ch. Coeff./1

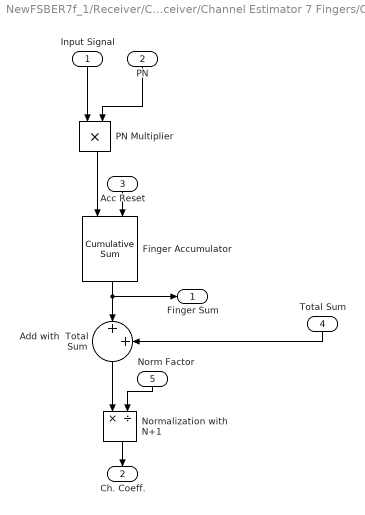
== system NewFSBER7f_1/Receiver/Channel Estimator and  Rake Receiver/Channel Estimator 7 Fingers/Channel Estimator Finger 4 ==
  Input Signal : Inport
  PN : Inport  Port=2
  Acc Reset : Inport  Port=3
  Total Sum : Inport  Port=4
  Norm Factor : Inport  Port=5
  Add with  Total Sum : Sum  Inputs=|++
  Finger Accumulator : dspmathops/Cumulative Sum  dim=Channels (running sum)  reset_popup=Rising edge  roundingMode=Floor  overflowMode=off
  Normalization with N+1 : Product  Inputs=*/
  PN Multiplier : Product  RndMeth=Zero
  Finger Sum : Outport
  Ch. Coeff. : Outport  Port=2
  wires:
  PN Multiplier/1 -> Finger Accumulator/1
  Finger Accumulator/1 -> Add with  Total Sum/1, Finger Sum/1
  Add with  Total Sum/1 -> Normalization with N+1/1
  Input Signal/1 -> PN Multiplier/1
  PN/1 -> PN Multiplier/2
  Acc Reset/1 -> Finger Accumulator/2
  Total Sum/1 -> Add with  Total Sum/2
  Norm Factor/1 -> Normalization with N+1/2
  Normalization with N+1/1 -> Ch. Coeff./1

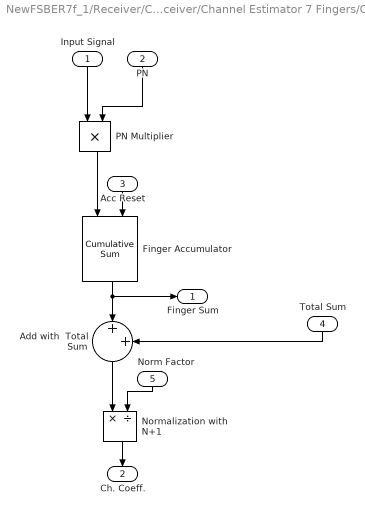
== system NewFSBER7f_1/Receiver/Channel Estimator and  Rake Receiver/Channel Estimator 7 Fingers/Channel Estimator Finger 5 ==
  Input Signal : Inport
  PN : Inport  Port=2
  Acc Reset : Inport  Port=3
  Total Sum : Inport  Port=4
  Norm Factor : Inport  Port=5
  Add with  Total Sum : Sum  Inputs=|++
  Finger Accumulator : dspmathops/Cumulative Sum  dim=Channels (running sum)  reset_popup=Rising edge  roundingMode=Floor  overflowMode=off
  Normalization with N+1 : Product  Inputs=*/
  PN Multiplier : Product  RndMeth=Zero
  Finger Sum : Outport
  Ch. Coeff. : Outport  Port=2
  wires:
  PN Multiplier/1 -> Finger Accumulator/1
  Finger Accumulator/1 -> Add with  Total Sum/1, Finger Sum/1
  Add with  Total Sum/1 -> Normalization with N+1/1
  Input Signal/1 -> PN Multiplier/1
  PN/1 -> PN Multiplier/2
  Acc Reset/1 -> Finger Accumulator/2
  Total Sum/1 -> Add with  Total Sum/2
  Norm Factor/1 -> Normalization with N+1/2
  Normalization with N+1/1 -> Ch. Coeff./1

== system NewFSBER7f_1/Receiver/Channel Estimator and  Rake Receiver/Channel Estimator 7 Fingers/Channel Estimator Finger 6 ==
  Input Signal : Inport
  PN : Inport  Port=2
  Acc Reset : Inport  Port=3
  Total Sum : Inport  Port=4
  Norm Factor : Inport  Port=5
  Add with  Total Sum : Sum  Inputs=|++
  Finger Accumulator : dspmathops/Cumulative Sum  dim=Channels (running sum)  reset_popup=Rising edge  roundingMode=Floor  overflowMode=off
  Normalization with N+1 : Product  Inputs=*/
  PN Multiplier : Product  RndMeth=Zero
  Finger Sum : Outport
  Ch. Coeff. : Outport  Port=2
  wires:
  PN Multiplier/1 -> Finger Accumulator/1
  Finger Accumulator/1 -> Add with  Total Sum/1, Finger Sum/1
  Add with  Total Sum/1 -> Normalization with N+1/1
  Input Signal/1 -> PN Multiplier/1
  PN/1 -> PN Multiplier/2
  Acc Reset/1 -> Finger Accumulator/2
  Total Sum/1 -> Add with  Total Sum/2
  Norm Factor/1 -> Normalization with N+1/2
  Normalization with N+1/1 -> Ch. Coeff./1

== system NewFSBER7f_1/Receiver/Channel Estimator and  Rake Receiver/Rake Receiver 7 Fingers/Rake Receiver Finger 0 ==
  Input Signal : Inport
  PN : Inport  Port=2
  Acc Reset : Inport  Port=3
  Channel Estimate : Inport  Port=4
  Finger Accumulator : dspmathops/Cumulative Sum  dim=Channels (running sum)  reset_popup=Rising edge  roundingMode=Floor  overflowMode=off
  Multiply with  Channel Estimate : Product  RndMeth=Zero
  PN Multiplier : Product  RndMeth=Zero
  Rake Component : Outport
  wires:
  PN Multiplier/1 -> Finger Accumulator/1
  Finger Accumulator/1 -> Multiply with  Channel Estimate/1
  Input Signal/1 -> PN Multiplier/1
  PN/1 -> PN Multiplier/2
  Acc Reset/1 -> Finger Accumulator/2
  Channel Estimate/1 -> Multiply with  Channel Estimate/2
  Multiply with  Channel Estimate/1 -> Rake Component/1

== system NewFSBER7f_1/Receiver/Channel Estimator and  Rake Receiver/Rake Receiver 7 Fingers/Rake Receiver Finger 1 ==
  Input Signal : Inport
  PN : Inport  Port=2
  Acc Reset : Inport  Port=3
  Channel Estimate : Inport  Port=4
  Finger Accumulator : dspmathops/Cumulative Sum  dim=Channels (running sum)  reset_popup=Rising edge  roundingMode=Floor  overflowMode=off
  Multiply with  Channel Estimate : Product  RndMeth=Zero
  PN Multiplier : Product  RndMeth=Zero
  Rake Component : Outport
  wires:
  Multiply with  Channel Estimate/1 -> Rake Component/1
  Channel Estimate/1 -> Multiply with  Channel Estimate/2
  Acc Reset/1 -> Finger Accumulator/2
  PN/1 -> PN Multiplier/2
  Input Signal/1 -> PN Multiplier/1
  Finger Accumulator/1 -> Multiply with  Channel Estimate/1
  PN Multiplier/1 -> Finger Accumulator/1

== system NewFSBER7f_1/Receiver/Channel Estimator and  Rake Receiver/Rake Receiver 7 Fingers/Rake Receiver Finger 2 ==
  Input Signal : Inport
  PN : Inport  Port=2
  Acc Reset : Inport  Port=3
  Channel Estimate : Inport  Port=4
  Finger Accumulator : dspmathops/Cumulative Sum  dim=Channels (running sum)  reset_popup=Rising edge  roundingMode=Floor  overflowMode=off
  Multiply with  Channel Estimate : Product  RndMeth=Zero
  PN Multiplier : Product  RndMeth=Zero
  Rake Component : Outport
  wires:
  PN Multiplier/1 -> Finger Accumulator/1
  Finger Accumulator/1 -> Multiply with  Channel Estimate/1
  Input Signal/1 -> PN Multiplier/1
  PN/1 -> PN Multiplier/2
  Acc Reset/1 -> Finger Accumulator/2
  Channel Estimate/1 -> Multiply with  Channel Estimate/2
  Multiply with  Channel Estimate/1 -> Rake Component/1

== system NewFSBER7f_1/Receiver/Channel Estimator and  Rake Receiver/Rake Receiver 7 Fingers/Rake Receiver Finger 3 ==
  Input Signal : Inport
  PN : Inport  Port=2
  Acc Reset : Inport  Port=3
  Channel Estimate : Inport  Port=4
  Finger Accumulator : dspmathops/Cumulative Sum  dim=Channels (running sum)  reset_popup=Rising edge  roundingMode=Floor  overflowMode=off
  Multiply with  Channel Estimate : Product  RndMeth=Zero
  PN Multiplier : Product  RndMeth=Zero
  Rake Component : Outport
  wires:
  Multiply with  Channel Estimate/1 -> Rake Component/1
  Channel Estimate/1 -> Multiply with  Channel Estimate/2
  Acc Reset/1 -> Finger Accumulator/2
  PN/1 -> PN Multiplier/2
  Input Signal/1 -> PN Multiplier/1
  Finger Accumulator/1 -> Multiply with  Channel Estimate/1
  PN Multiplier/1 -> Finger Accumulator/1

== system NewFSBER7f_1/Receiver/Channel Estimator and  Rake Receiver/Rake Receiver 7 Fingers/Rake Receiver Finger 4 ==
  Input Signal : Inport
  PN : Inport  Port=2
  Acc Reset : Inport  Port=3
  Channel Estimate : Inport  Port=4
  Finger Accumulator : dspmathops/Cumulative Sum  dim=Channels (running sum)  reset_popup=Rising edge  roundingMode=Floor  overflowMode=off
  Multiply with  Channel Estimate : Product  RndMeth=Zero
  PN Multiplier : Product  RndMeth=Zero
  Rake Component : Outport
  wires:
  PN Multiplier/1 -> Finger Accumulator/1
  Finger Accumulator/1 -> Multiply with  Channel Estimate/1
  Input Signal/1 -> PN Multiplier/1
  PN/1 -> PN Multiplier/2
  Acc Reset/1 -> Finger Accumulator/2
  Channel Estimate/1 -> Multiply with  Channel Estimate/2
  Multiply with  Channel Estimate/1 -> Rake Component/1

== system NewFSBER7f_1/Receiver/Channel Estimator and  Rake Receiver/Rake Receiver 7 Fingers/Rake Receiver Finger 5 ==
  Input Signal : Inport
  PN : Inport  Port=2
  Acc Reset : Inport  Port=3
  Channel Estimate : Inport  Port=4
  Finger Accumulator : dspmathops/Cumulative Sum  dim=Channels (running sum)  reset_popup=Rising edge  roundingMode=Floor  overflowMode=off
  Multiply with  Channel Estimate : Product  RndMeth=Zero
  PN Multiplier : Product  RndMeth=Zero
  Rake Component : Outport
  wires:
  Multiply with  Channel Estimate/1 -> Rake Component/1
  Channel Estimate/1 -> Multiply with  Channel Estimate/2
  Acc Reset/1 -> Finger Accumulator/2
  PN/1 -> PN Multiplier/2
  Input Signal/1 -> PN Multiplier/1
  Finger Accumulator/1 -> Multiply with  Channel Estimate/1
  PN Multiplier/1 -> Finger Accumulator/1

== system NewFSBER7f_1/Receiver/Channel Estimator and  Rake Receiver/Rake Receiver 7 Fingers/Rake Receiver Finger 6 ==
  Input Signal : Inport
  PN : Inport  Port=2
  Acc Reset : Inport  Port=3
  Channel Estimate : Inport  Port=4
  Finger Accumulator : dspmathops/Cumulative Sum  dim=Channels (running sum)  reset_popup=Rising edge  roundingMode=Floor  overflowMode=off
  Multiply with  Channel Estimate : Product  RndMeth=Zero
  PN Multiplier : Product  RndMeth=Zero
  Rake Component : Outport
  wires:
  PN Multiplier/1 -> Finger Accumulator/1
  Finger Accumulator/1 -> Multiply with  Channel Estimate/1
  Input Signal/1 -> PN Multiplier/1
  PN/1 -> PN Multiplier/2
  Acc Reset/1 -> Finger Accumulator/2
  Channel Estimate/1 -> Multiply with  Channel Estimate/2
  Multiply with  Channel Estimate/1 -> Rake Component/1
